simulink model "tesis_entrenador"  (R2013a)
settings: Solver=VariableStepDiscrete  StartTime=0.0  StopTime=100000  FixedStep=1  MaxStep=1  RelTol=1e-3
model workspace (MAT data in the model file):
  i = 1
libraries: simulink x1, commfilt2 x1
settings Model: Creator=marcos  LastModifiedBy=marcos

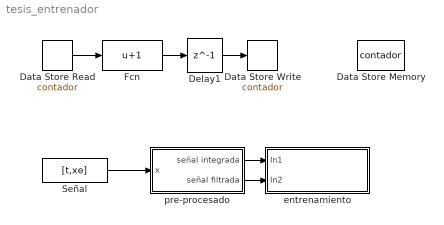
== system tesis_entrenador ==
  Data Store Memory : DataStoreMemory  DataStoreName=contador  ReadBeforeWriteMsg=warning  WriteAfterWriteMsg=warning  WriteAfterReadMsg=warning  InitialValue=1  OutDataTypeStr=double  Dimensions=1
  Data Store Read : DataStoreRead  DataStoreName=contador  SampleTime=1  DataStoreElements=contador
  Data Store Write : DataStoreWrite  DataStoreName=contador  SampleTime=1  DataStoreElements=contador
  Delay1 : Delay  DelayLength=1  InitialCondition=0  SampleTime=1
  Fcn : Fcn  Expr=u+1  SampleTime=1
  Señal : FromWorkspace  VariableName=[t,xe]  SampleTime=1
  entrenamiento : Subsystem
  pre-procesado : Subsystem
  wires:
  Señal/1 -> pre-procesado/1(x)
  pre-procesado/1(señal integrada) -> entrenamiento/1(In1)
  Fcn/1 -> Delay1/1
  Data Store Read/1 -> Fcn/1
  pre-procesado/2(señal filtrada) -> entrenamiento/2(In2)
  Delay1/1 -> Data Store Write/1

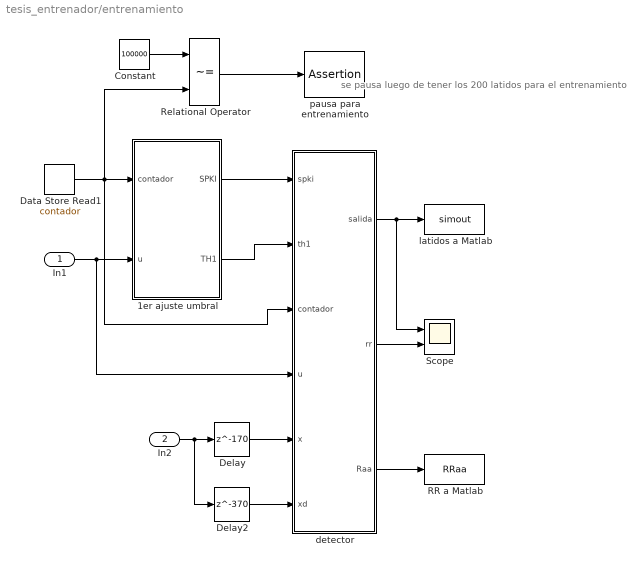
== system tesis_entrenador/entrenamiento ==
  note: se pausa luego de tener los 200
      | latidos para el entrenamiento
  In1 : Inport
  In2 : Inport  Port=2
  1er ajuste umbral : MATLAB Function  TreatAsAtomicUnit=on
  Constant : Constant  Value=100000
  Data Store Read1 : DataStoreRead  DataStoreName=contador  SampleTime=1
  Delay : Delay  DelayLength=170  InitialCondition=0  SampleTime=1
  Delay2 : Delay  DelayLength=370  InitialCondition=0  SampleTime=1
  RR a Matlab : ToWorkspace  VariableName=RRaa  SampleTime=1
  Relational Operator : RelationalOperator  Operator=~=  OutDataTypeStr=boolean  SampleTime=1
  Scope : Scope  NumInputPorts=2
      settings: TimeRange=10000  YMin=-40~0.8500000000000001  YMax=80~1.25  MaxDataPoints=10000
  detector : MATLAB Function  TreatAsAtomicUnit=on
  latidos a Matlab : ToWorkspace  VariableName=simout  SampleTime=-1
  pausa para entrenamiento : Assertion  AssertionFailFcn=|  StopWhenAssertionFail=off  SampleTime=1
      | set_param(bdroot,'SimulationCommand','pause'),
      | disp(sprintf('\nSimulation paused.'))
  wires:
  In1/1 -> detector/4(u), 1er ajuste umbral/2(u)
  Data Store Read1/1 -> Relational Operator/2, detector/3(contador), 1er ajuste umbral/1(contador)
  1er ajuste umbral/1(SPKI) -> detector/1(spki)
  1er ajuste umbral/2(TH1) -> detector/2(th1)
  In2/1 -> Delay/1, Delay2/1
  detector/1(salida) -> Scope/1, latidos a Matlab/1
  Delay2/1 -> detector/6(xd)
  Delay/1 -> detector/5(x)
  Constant/1 -> Relational Operator/1
  Relational Operator/1 -> pausa para entrenamiento/1
  detector/2(rr) -> Scope/2
  detector/3(Raa) -> RR a Matlab/1

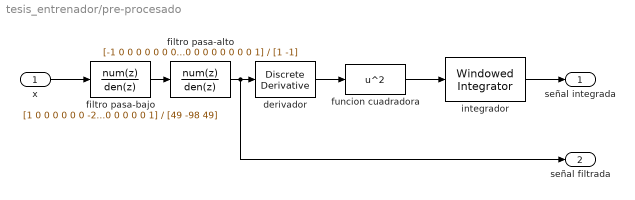
== system tesis_entrenador/pre-procesado ==
  x : Inport
  derivador : simulink/Discrete/Discrete Derivative  gainval=1.0  ICPrevScaledInput=0.0  InputProcessing=Inherited  OutMin=[]  OutMax=[]  OutDataType=fixdt(1, 16)  OutScaling=2^-10  DoSatur=off
  filtro pasa-alto : DiscreteFilter  Numerator=[-1 0 0 0 0 0 0 0 0 0 0 0 0 0 0 0 0 0 0 0 0 0 0 0 48 -48 0 0 0 0 0 0 0 0 0 0 0 0 0 0 0 0 0 0 0 0 0 0 1]  Denominator=[1 -1]
  filtro pasa-bajo : DiscreteFilter  Numerator=[1 0 0 0 0 0 0 -2 0 0 0 0 0 0 1]  Denominator=[49 -98 49]
  funcion cuadradora : Fcn  Expr=u^2
  integrador : commfilt2/Windowed Integrator  integperiod=64  roundingMode=Floor  overflowMode=off
  señal integrada : Outport
  señal filtrada : Outport  Port=2
  wires:
  x/1 -> filtro pasa-bajo/1
  filtro pasa-bajo/1 -> filtro pasa-alto/1
  filtro pasa-alto/1 -> señal filtrada/1, derivador/1
  derivador/1 -> funcion cuadradora/1
  funcion cuadradora/1 -> integrador/1
  integrador/1 -> señal integrada/1

== matlab function tesis_entrenador/entrenamiento/detector ==
  data: spki input; th1 input; contador input; u input; salida output; x input; rr output; xd input; Raa output
function [salida,rr,Raa]= fcn(spki,th1,contador,u,x,xd) 
%#codegen

%se definen las variables
persistent peak;
persistent TH1;
persistent SPKI;
persistent NPKI;
persistent bandera;     %bandera para buscar loma (1) o detectar qrs (2)
persistent guardar;     %bandera para guardar
persistent cuenta;
persistent sal;
persistent m_anterior;  %muestra anterior
persistent x_max;
persistent index;
persistent save;
persistent cuen;
persistent bkRR;
persistent relacion;
persistent relacion2;
persistent pos_pico;

%se inician las variables
if isempty(peak)
    bkRR=[nan nan nan];
    peak=0;
    TH1=0;
    cuenta=1;
    guardar=0;
    sal=nan;
    m_anterior=-5;
    x_max=-10;
    bandera=1;
    index=nan;
    save=0;
    cuen=1;
    relacion=nan;
    relacion2=nan;
    pos_pico=nan;
end



%empiezo a detectar dsp del primer segundo 
if contador > 360

if isempty(SPKI)
    TH1=th1;
    NPKI=0;
    SPKI=spki;
end

switch (bandera)
    case {1} %Buscador de loma
        if u > m_anterior
            peak=u;
            bandera=2;
        end
        
    case {2} %Detector de QRS
        
        if u < (peak/2)

            if peak > TH1
            %actualiacion del umbral adaptativo (debido a la señal)
            SPKI=0.125*peak+0.875*SPKI;
            
            bandera=0;
            cuenta=1;
            guardar=1;
                        
            else
            %actualiacion del umbral adaptativo (debido al ruido)
            NPKI=0.125*peak+0.875*NPKI;
            bandera=1;
            end
            
        %actualiacion del umbral adaptativo
        TH1=NPKI+0.21*(SPKI-NPKI);
                
        
        elseif u > peak
        
        peak=u;
        
        end
    
    sal=nan;
    
end
        
%busco pico R
relacion=nan;
relacion2=nan;

if guardar==1
    if cuenta <= 200
        if x > x_max
            index=cuenta;
            x_max=x;
            pos_pico=contador;
        end
        
    else
        %guardo los RR
        bkRR(3)=bkRR(2);
        bkRR(2)=bkRR(1);
        bkRR(1)=pos_pico;
        
        relacion=(bkRR(1)-bkRR(2))/(bkRR(2)-bkRR(3));
        relacion2=relacion;
        
        save=1;
        x_max=-10;
        guardar=0;
        bandera=1;
        cuen=1;
        
    end

    cuenta=cuenta+1;
end

%guarda el latido centrado en R
if save==1
    if cuen >= (index-100) && cuen <= (index+100)
        
        sal=xd;
        relacion=(bkRR(1)-bkRR(2))/(bkRR(2)-bkRR(3));
        
    elseif cuen == (100+index)
        save=0;
        cuen=0;
        
    end

    cuen=cuen+1;
end

end
%guardo el valor actual para usarlo en el paso siguiente
m_anterior=u;

clasif=index;
t=TH1;
p=peak;
salida=sal;
rr=relacion;
Raa=relacion2;

== matlab function tesis_entrenador/entrenamiento/1er ajuste umbral ==
  data: contador input; u input; SPKI output; TH1 output
function [SPKI,TH1]= fcn(contador,u) 
%#codegen
persistent peak

if isempty(peak)
    peak=0;
end

if contador < 360

    if u > peak
        peak=u;
    end

end

%Ajuste de los umbrales de deteccion
%SPKI es el estimado del pico de señal
%NPKI es el estimado del pico de ruido
%THRESHOLD1 es el primer umbral aplicado 
%THRESHOLD2 es el segundo umbral aplicado.
SPKI=peak/2;
SPKI=0.125*peak+0.875*SPKI;

TH1=peak/4;

end
